simulink model "ABSOLUTE_ENCODER"  (R2019b)
settings: Solver=VariableStepAuto  StartTime=0.0  StopTime=10.0  RelTol=1e-3
libraries: hdlsllib x13, simulink_extras x3
settings Model: Creator=simone  LastModifiedBy=simone

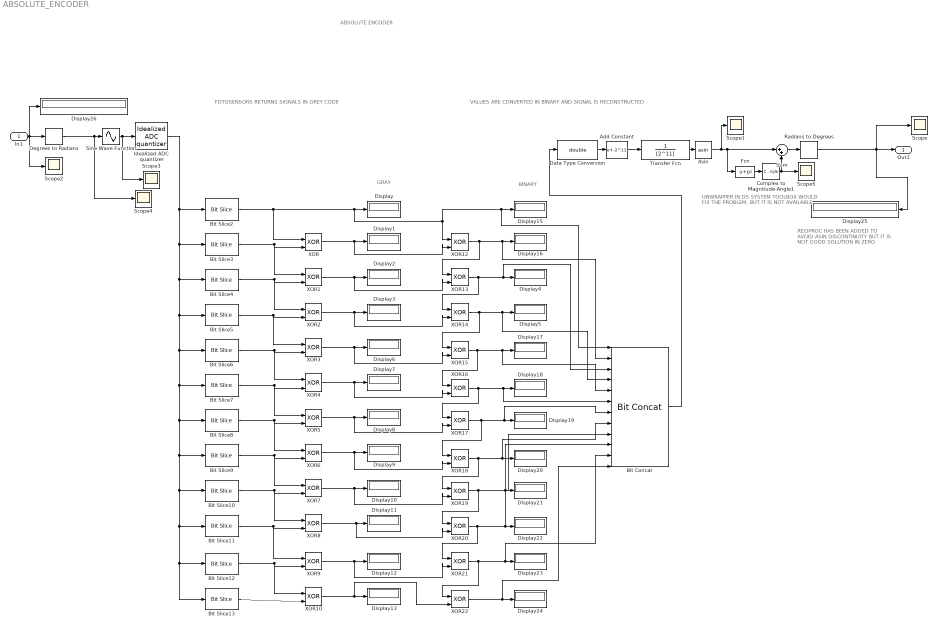
== system ABSOLUTE_ENCODER ==
  note: RECIPROC HAS BEEN ADDED
      | TO AVOID ASIN DISCONTINUITY
      | BUT IT IS NOT GOOD SOLUTION
      | IN ZERO
  note: VALUES ARE CONVERTED IN BINARY
      | AND SIGNAL IS RECONSTRUCTED
  note: BINARY
  note: GRAY
  note: ABSOLUTE ENCODER
  note: FOTOSENSORS RETURNS
      | SIGNALS IN GREY CODE
  note: UNWRAPPER IN DS SYSTEM TOOLBOX
      | WOULD FIX THE PROBLEM, BUT IT IS
      | NOT AVAILABLE
  In1 : Inport
  Add Constant : Bias  Bias=-2^11
  Asin : Trigonometry  Operator=asin
  Bit Concat : hdlsllib/Logic and Bit Operations/Bit Concat  numInputs=12
      settings: SourceProductName=Simulink
  Bit Slice10 : hdlsllib/Logic and Bit Operations/Bit Slice  lidx=3  ridx=3
      settings: SourceProductName=Simulink  SourceProductBaseCode=SL
  Bit Slice11 : hdlsllib/Logic and Bit Operations/Bit Slice  lidx=2  ridx=2
      settings: SourceProductName=Simulink  SourceProductBaseCode=SL
  Bit Slice12 : hdlsllib/Logic and Bit Operations/Bit Slice  lidx=1  ridx=1
      settings: SourceProductName=Simulink  SourceProductBaseCode=SL
  Bit Slice13 : hdlsllib/Logic and Bit Operations/Bit Slice  lidx=0  ridx=0
      settings: SourceProductName=Simulink  SourceProductBaseCode=SL
  Bit Slice2 : hdlsllib/Logic and Bit Operations/Bit Slice  lidx=11  ridx=11
      settings: SourceProductName=Simulink  SourceProductBaseCode=SL
  Bit Slice3 : hdlsllib/Logic and Bit Operations/Bit Slice  lidx=10  ridx=10
      settings: SourceProductName=Simulink  SourceProductBaseCode=SL
  Bit Slice4 : hdlsllib/Logic and Bit Operations/Bit Slice  lidx=9  ridx=9
      settings: SourceProductName=Simulink  SourceProductBaseCode=SL
  Bit Slice5 : hdlsllib/Logic and Bit Operations/Bit Slice  lidx=8  ridx=8
      settings: SourceProductName=Simulink  SourceProductBaseCode=SL
  Bit Slice6 : hdlsllib/Logic and Bit Operations/Bit Slice  lidx=7  ridx=7
      settings: SourceProductName=Simulink  SourceProductBaseCode=SL
  Bit Slice7 : hdlsllib/Logic and Bit Operations/Bit Slice  lidx=6  ridx=6
      settings: SourceProductName=Simulink  SourceProductBaseCode=SL
  Bit Slice8 : hdlsllib/Logic and Bit Operations/Bit Slice  lidx=5  ridx=5
      settings: SourceProductName=Simulink  SourceProductBaseCode=SL
  Bit Slice9 : hdlsllib/Logic and Bit Operations/Bit Slice  lidx=4  ridx=4
      settings: SourceProductName=Simulink  SourceProductBaseCode=SL
  Complex to Magnitude-Angle1 : ComplexToMagnitudeAngle  Output=Angle
  Data Type Conversion : DataTypeConversion  OutDataTypeStr=double
  Degrees to Radians : simulink_extras/Transformations/Degrees to Radians
  Display{,1..13,15..26} (26 alike) : Display
  Fcn : Fcn  Expr=u+pi
  Idealized ADC quantizer : simulink_extras/Additional Discrete/Idealized ADC quantizer  NumberOfConverterBits=12  Vmin=-1  Vmax=1  OutputDataType=uint16  OutputNegativeValues=off
      settings: SourceProductName=Simulink
  Radians to Degrees : simulink_extras/Transformations/Radians to Degrees
  Scope{,1..5} (6 alike) : Scope
  Sine Wave Function : Sin  TimeSource=Use external signal  SampleTime=0
  Sum : Sum  Inputs=|++
  Transfer Fcn : TransferFcn  Denominator=[2^11]
  XOR{,1..10,12..22} (22 alike) : Logic  Operator=XOR  IconShape=distinctive  AllPortsSameDT=off  OutDataTypeStr=boolean
  Out1 : Outport
  wires:
  Bit Slice4/1 -> XOR2/1, XOR1/2
  Bit Slice3/1 -> XOR1/1, XOR/2
  In1/1 -> Scope2/1, Display26/1, Degrees to Radians/1
  Sine Wave Function/1 -> Scope3/1, Idealized ADC quantizer/1
  Bit Slice7/1 -> XOR5/1, XOR4/2
  Bit Slice5/1 -> XOR3/1, XOR2/2
  Bit Slice6/1 -> XOR4/1, XOR3/2
  Bit Slice10/1 -> XOR8/1, XOR7/2
  Bit Slice8/1 -> XOR6/1, XOR5/2
  Bit Slice9/1 -> XOR7/1, XOR6/2
  Bit Slice11/1 -> XOR9/1, XOR8/2
  Bit Slice12/1 -> XOR10/1, XOR9/2
  Bit Slice13/1 -> XOR10/2
  XOR2/1 -> XOR14/2, Display3/1
  XOR/1 -> XOR12/2, Display1/1
  XOR12/1 -> XOR13/1, Bit Concat/2, Display16/1
  XOR1/1 -> XOR13/2, Display2/1
  XOR3/1 -> XOR15/2, Display6/1
  XOR15/1 -> XOR16/1, Bit Concat/5, Display17/1
  XOR4/1 -> XOR16/2, Display7/1
  XOR16/1 -> XOR17/1, Bit Concat/6, Display18/1
  XOR5/1 -> XOR17/2, Display8/1
  XOR17/1 -> XOR18/1, Bit Concat/7, Display19/1
  XOR6/1 -> XOR18/2, Display9/1
  XOR18/1 -> XOR19/1, Bit Concat/8, Display20/1
  XOR7/1 -> XOR19/2, Display10/1
  XOR19/1 -> XOR20/1, Bit Concat/9, Display21/1
  XOR8/1 -> XOR20/2, Display11/1
  XOR20/1 -> XOR21/1, Bit Concat/10, Display22/1
  XOR9/1 -> XOR21/2, Display12/1
  XOR21/1 -> XOR22/1, Bit Concat/11, Display23/1
  XOR10/1 -> XOR22/2, Display13/1
  Bit Slice2/1 -> XOR/1, Display/1, XOR12/1, Display15/1, Bit Concat/1
  XOR13/1 -> XOR14/1, Bit Concat/3, Display4/1
  XOR14/1 -> XOR15/1, Bit Concat/4, Display5/1
  XOR22/1 -> Bit Concat/12, Display24/1
  Bit Concat/1 -> Data Type Conversion/1
  Data Type Conversion/1 -> Add Constant/1
  Add Constant/1 -> Transfer Fcn/1
  Idealized ADC quantizer/1 -> Bit Slice2/1, Bit Slice3/1, Bit Slice4/1, Bit Slice5/1, Bit Slice6/1, Bit Slice7/1, Bit Slice8/1, Bit Slice9/1, Bit Slice10/1, Bit Slice11/1, Bit Slice12/1, Bit Slice13/1
  Transfer Fcn/1 -> Asin/1
  Degrees to Radians/1 -> Scope4/1, Sine Wave Function/1
  Asin/1 -> Fcn/1, Sum/1, Scope1/1
  Radians to Degrees/1 -> Out1/1, Display25/1, Scope/1
  Sum/1 -> Radians to Degrees/1
  Complex to Magnitude-Angle1/1 -> Sum/2, Scope5/1
  Fcn/1 -> Complex to Magnitude-Angle1/1
